simulink model "building_PHPP_carnot83"  (R2023b)
settings: Solver=ode23s  StartTime=-building.preruntime+8760*3600  StopTime=building.runtime+8760*3600  EnableMultiTasking=on
StartFcn:
  | tic
StopFcn:
  | toc
values from neighbouring files (symbols this model uses):
  building = obj    [BUILDING.m]    (also in create_building_automatic.m = building.save(); ini_building_automatic.m = building.add_variant_hvac(building.variant_hvac, hvac); load_building_automatic.m = building.save())
  cp = str2num(value)    [CONSTRUCTION.m]
  p = [timevec_weather weather(:,12)]    [BOUNDARY.m]    (also in WEATHER.m = 0; init_carnotUIBK.m = cell2mat(carnotUIBKpaths(i,2)))
  rho = str2num(value)    [CONSTRUCTION.m]    (also in theta_ground_v1.m = 2000)
undefined symbols (not defined in the file or in its folder): Dreifach, get_building, Qdot_C, Qdot_C_energy, Qdot_H, Qdot_H_energy, Qdot_I_electricity, Qdot_I_electricity_energy, Qdot_I_light, Qdot_I_light_energy, Qdot_I_person, Qdot_I_person_energy, Qdot_S, Qdot_S_energy, Qdot_T_ground, Qdot_T_ground_energy, Qdot_T_neighbour, Qdot_T_neighbour_energy, Qdot_T_opaque, Qdot_T_opaque_energy, Qdot_T_window, Qdot_T_window_energy, Qdot_V_infiltration, Qdot_V_infiltration_energy, Qdot_V_mech, Qdot_V_mech_energy, Qdot_V_window, Qdot_V_window_energy, Tc, Tr, Ts, Wärmeschutzglas, x_CO2, x_H2O, x_VOC
libraries: carnotUIBK x2418, carnot x1
(part 5 of 32)

== system building_PHPP_carnot83/BUILDING/INTERSECTION_7_9 ==
  AIB1 : Inport
  AIB2 : Inport  Port=2
  BDB1 : Inport  Port=3
  BDB2 : Inport  Port=4
  control : Inport  Port=5
  Bus Selector : BusSelector  OutputSignals=Qdot_S
  Bus Selector1 : BusSelector  OutputSignals=Qdot_S
  Subsystem : Subsystem
  Subsystem1 : Subsystem
  airexchange_1 : Subsystem  Variant=on  mask{zone=i.matrix_wd, window=1}
      mask prompts: window "wall"
      mask init: same as building_PHPP_carnot83/BUILDING/INTERSECTION_1_10/airexchange_1
      mask Display:
      | fprintf('AIR EXCHANGE\n')
      | %fprintf('\n%s', const.name)
  airexchange_2 : Subsystem  Variant=on  mask{zone=i.matrix_wd, window=2}
      mask prompts: window "wall"
      mask init: same as building_PHPP_carnot83/BUILDING/INTERSECTION_1_10/airexchange_1
      mask Display:
      | fprintf('AIR EXCHANGE\n')
      | %fprintf('\n%s', const.name)
  airexchange_3 : Subsystem  Variant=on  mask{zone=i.matrix_wd, window=3}
      mask prompts: window "wall"
      mask init: same as building_PHPP_carnot83/BUILDING/INTERSECTION_1_10/airexchange_1
      mask Display:
      | fprintf('AIR EXCHANGE\n')
      | %fprintf('\n%s', const.name)
  wall_1 : Subsystem  Variant=on  mask{zone=i.matrix_wd, construction=b.construction, wall=1}
      mask init: same as building_PHPP_carnot83/BUILDING/INTERSECTION_1_10/wall_1
      mask Display:
      | fprintf('CONSTRUCTION:\n')
      | fprintf('\n%s', const.name)
  wall_2 : Subsystem  Variant=on  mask{zone=i.matrix_wd, construction=b.construction, wall=2}
      mask init: same as building_PHPP_carnot83/BUILDING/INTERSECTION_1_10/wall_1
      mask Display:
      | fprintf('CONSTRUCTION:\n')
      | fprintf('\n%s', const.name)
  wall_3 : Subsystem  Variant=on  mask{zone=i.matrix_wd, construction=b.construction, wall=3}
      mask init: same as building_PHPP_carnot83/BUILDING/INTERSECTION_1_10/wall_1
      mask Display:
      | fprintf('CONSTRUCTION:\n')
      | fprintf('\n%s', const.name)
  S1 : Outport  VectorParamsAs1DForOutWhenUnconnected=off
  S2 : Outport  Port=2  VectorParamsAs1DForOutWhenUnconnected=off
  wires:
  BDB1/1 -> Bus Selector/1
  Bus Selector/1 -> wall_1/3(Qdot_sol1), wall_2/3(Qdot_sol1), wall_3/3(Qdot_sol1)  "<Qdot_S>"
  BDB2/1 -> Bus Selector1/1
  Bus Selector1/1 -> wall_1/4(Qdot_sol2), wall_2/4(Qdot_sol2), wall_3/4(Qdot_sol2)  "<Qdot_S>"
  control/1 -> airexchange_3/3(control), airexchange_2/3(control), airexchange_1/3(control)
  AIB2/1 -> wall_2/2(AIB2), wall_3/2(AIB2), airexchange_3/2(AIB2), airexchange_2/2(AIB2), airexchange_1/2(AIB2), wall_1/2(AIB2)
  AIB1/1 -> wall_2/1(AIB1), wall_3/1(AIB1), airexchange_3/1(AIB1), airexchange_2/1(AIB1), airexchange_1/1(AIB1), wall_1/1(AIB1)
  wall_1/1("[S1]") -> Subsystem/1(S1)
  wall_2/1("[S1]") -> Subsystem/2(S2)
  wall_3/1("[S1]") -> Subsystem/3(S3)
  airexchange_1/1("[S1]") -> Subsystem/4(S4)
  airexchange_2/1("[S1]") -> Subsystem/5(S5)
  airexchange_3/1("[S1]") -> Subsystem/6(S6)
  wall_1/2("[S2]") -> Subsystem1/1(S1)
  wall_2/2("[S2]") -> Subsystem1/2(S2)
  airexchange_3/2("[S2]") -> Subsystem1/6(S6)
  airexchange_2/2("[S2]") -> Subsystem1/5(S5)
  airexchange_1/2("[S2]") -> Subsystem1/4(S4)
  wall_3/2("[S2]") -> Subsystem1/3(S3)
  Subsystem/1(Sout) -> S1/1
  Subsystem1/1(Sout) -> S2/1

== system building_PHPP_carnot83/BUILDING/INTERSECTION_8_10 ==
  AIB1 : Inport
  AIB2 : Inport  Port=2
  BDB1 : Inport  Port=3
  BDB2 : Inport  Port=4
  control : Inport  Port=5
  Bus Selector : BusSelector  OutputSignals=Qdot_S
  Bus Selector1 : BusSelector  OutputSignals=Qdot_S
  Subsystem : Subsystem
  Subsystem1 : Subsystem
  airexchange_1 : Subsystem  Variant=on  mask{zone=i.matrix_wd, window=1}
      mask prompts: window "wall"
      mask init: same as building_PHPP_carnot83/BUILDING/INTERSECTION_1_10/airexchange_1
      mask Display:
      | fprintf('AIR EXCHANGE\n')
      | %fprintf('\n%s', const.name)
  airexchange_2 : Subsystem  Variant=on  mask{zone=i.matrix_wd, window=2}
      mask prompts: window "wall"
      mask init: same as building_PHPP_carnot83/BUILDING/INTERSECTION_1_10/airexchange_1
      mask Display:
      | fprintf('AIR EXCHANGE\n')
      | %fprintf('\n%s', const.name)
  airexchange_3 : Subsystem  Variant=on  mask{zone=i.matrix_wd, window=3}
      mask prompts: window "wall"
      mask init: same as building_PHPP_carnot83/BUILDING/INTERSECTION_1_10/airexchange_1
      mask Display:
      | fprintf('AIR EXCHANGE\n')
      | %fprintf('\n%s', const.name)
  wall_1 : Subsystem  Variant=on  mask{zone=i.matrix_wd, construction=b.construction, wall=1}
      mask init: same as building_PHPP_carnot83/BUILDING/INTERSECTION_1_10/wall_1
      mask Display:
      | fprintf('CONSTRUCTION:\n')
      | fprintf('\n%s', const.name)
  wall_2 : Subsystem  Variant=on  mask{zone=i.matrix_wd, construction=b.construction, wall=2}
      mask init: same as building_PHPP_carnot83/BUILDING/INTERSECTION_1_10/wall_1
      mask Display:
      | fprintf('CONSTRUCTION:\n')
      | fprintf('\n%s', const.name)
  wall_3 : Subsystem  Variant=on  mask{zone=i.matrix_wd, construction=b.construction, wall=3}
      mask init: same as building_PHPP_carnot83/BUILDING/INTERSECTION_1_10/wall_1
      mask Display:
      | fprintf('CONSTRUCTION:\n')
      | fprintf('\n%s', const.name)
  S1 : Outport  VectorParamsAs1DForOutWhenUnconnected=off
  S2 : Outport  Port=2  VectorParamsAs1DForOutWhenUnconnected=off
  wires:
  BDB1/1 -> Bus Selector/1
  Bus Selector/1 -> wall_1/3(Qdot_sol1), wall_2/3(Qdot_sol1), wall_3/3(Qdot_sol1)  "<Qdot_S>"
  BDB2/1 -> Bus Selector1/1
  Bus Selector1/1 -> wall_1/4(Qdot_sol2), wall_2/4(Qdot_sol2), wall_3/4(Qdot_sol2)  "<Qdot_S>"
  control/1 -> airexchange_3/3(control), airexchange_2/3(control), airexchange_1/3(control)
  AIB2/1 -> wall_2/2(AIB2), wall_3/2(AIB2), airexchange_3/2(AIB2), airexchange_2/2(AIB2), airexchange_1/2(AIB2), wall_1/2(AIB2)
  AIB1/1 -> wall_2/1(AIB1), wall_3/1(AIB1), airexchange_3/1(AIB1), airexchange_2/1(AIB1), airexchange_1/1(AIB1), wall_1/1(AIB1)
  wall_1/1("[S1]") -> Subsystem/1(S1)
  wall_2/1("[S1]") -> Subsystem/2(S2)
  wall_3/1("[S1]") -> Subsystem/3(S3)
  airexchange_1/1("[S1]") -> Subsystem/4(S4)
  airexchange_2/1("[S1]") -> Subsystem/5(S5)
  airexchange_3/1("[S1]") -> Subsystem/6(S6)
  wall_1/2("[S2]") -> Subsystem1/1(S1)
  wall_2/2("[S2]") -> Subsystem1/2(S2)
  airexchange_3/2("[S2]") -> Subsystem1/6(S6)
  airexchange_2/2("[S2]") -> Subsystem1/5(S5)
  airexchange_1/2("[S2]") -> Subsystem1/4(S4)
  wall_3/2("[S2]") -> Subsystem1/3(S3)
  Subsystem/1(Sout) -> S1/1
  Subsystem1/1(Sout) -> S2/1

== system building_PHPP_carnot83/BUILDING/INTERSECTION_8_9 ==
  AIB1 : Inport
  AIB2 : Inport  Port=2
  BDB1 : Inport  Port=3
  BDB2 : Inport  Port=4
  control : Inport  Port=5
  Bus Selector : BusSelector  OutputSignals=Qdot_S
  Bus Selector1 : BusSelector  OutputSignals=Qdot_S
  Subsystem : Subsystem
  Subsystem1 : Subsystem
  airexchange_1 : Subsystem  Variant=on  mask{zone=i.matrix_wd, window=1}
      mask prompts: window "wall"
      mask init: same as building_PHPP_carnot83/BUILDING/INTERSECTION_1_10/airexchange_1
      mask Display:
      | fprintf('AIR EXCHANGE\n')
      | %fprintf('\n%s', const.name)
  airexchange_2 : Subsystem  Variant=on  mask{zone=i.matrix_wd, window=2}
      mask prompts: window "wall"
      mask init: same as building_PHPP_carnot83/BUILDING/INTERSECTION_1_10/airexchange_1
      mask Display:
      | fprintf('AIR EXCHANGE\n')
      | %fprintf('\n%s', const.name)
  airexchange_3 : Subsystem  Variant=on  mask{zone=i.matrix_wd, window=3}
      mask prompts: window "wall"
      mask init: same as building_PHPP_carnot83/BUILDING/INTERSECTION_1_10/airexchange_1
      mask Display:
      | fprintf('AIR EXCHANGE\n')
      | %fprintf('\n%s', const.name)
  wall_1 : Subsystem  Variant=on  mask{zone=i.matrix_wd, construction=b.construction, wall=1}
      mask init: same as building_PHPP_carnot83/BUILDING/INTERSECTION_1_10/wall_1
      mask Display:
      | fprintf('CONSTRUCTION:\n')
      | fprintf('\n%s', const.name)
  wall_2 : Subsystem  Variant=on  mask{zone=i.matrix_wd, construction=b.construction, wall=2}
      mask init: same as building_PHPP_carnot83/BUILDING/INTERSECTION_1_10/wall_1
      mask Display:
      | fprintf('CONSTRUCTION:\n')
      | fprintf('\n%s', const.name)
  wall_3 : Subsystem  Variant=on  mask{zone=i.matrix_wd, construction=b.construction, wall=3}
      mask init: same as building_PHPP_carnot83/BUILDING/INTERSECTION_1_10/wall_1
      mask Display:
      | fprintf('CONSTRUCTION:\n')
      | fprintf('\n%s', const.name)
  S1 : Outport  VectorParamsAs1DForOutWhenUnconnected=off
  S2 : Outport  Port=2  VectorParamsAs1DForOutWhenUnconnected=off
  wires:
  BDB1/1 -> Bus Selector/1
  Bus Selector/1 -> wall_1/3(Qdot_sol1), wall_2/3(Qdot_sol1), wall_3/3(Qdot_sol1)  "<Qdot_S>"
  BDB2/1 -> Bus Selector1/1
  Bus Selector1/1 -> wall_1/4(Qdot_sol2), wall_2/4(Qdot_sol2), wall_3/4(Qdot_sol2)  "<Qdot_S>"
  control/1 -> airexchange_3/3(control), airexchange_2/3(control), airexchange_1/3(control)
  AIB2/1 -> wall_2/2(AIB2), wall_3/2(AIB2), airexchange_3/2(AIB2), airexchange_2/2(AIB2), airexchange_1/2(AIB2), wall_1/2(AIB2)
  AIB1/1 -> wall_2/1(AIB1), wall_3/1(AIB1), airexchange_3/1(AIB1), airexchange_2/1(AIB1), airexchange_1/1(AIB1), wall_1/1(AIB1)
  wall_1/1("[S1]") -> Subsystem/1(S1)
  wall_2/1("[S1]") -> Subsystem/2(S2)
  wall_3/1("[S1]") -> Subsystem/3(S3)
  airexchange_1/1("[S1]") -> Subsystem/4(S4)
  airexchange_2/1("[S1]") -> Subsystem/5(S5)
  airexchange_3/1("[S1]") -> Subsystem/6(S6)
  wall_1/2("[S2]") -> Subsystem1/1(S1)
  wall_2/2("[S2]") -> Subsystem1/2(S2)
  airexchange_3/2("[S2]") -> Subsystem1/6(S6)
  airexchange_2/2("[S2]") -> Subsystem1/5(S5)
  airexchange_1/2("[S2]") -> Subsystem1/4(S4)
  wall_3/2("[S2]") -> Subsystem1/3(S3)
  Subsystem/1(Sout) -> S1/1
  Subsystem1/1(Sout) -> S2/1

== system building_PHPP_carnot83/BUILDING/INTERSECTION_9_10 ==
  AIB1 : Inport
  AIB2 : Inport  Port=2
  BDB1 : Inport  Port=3
  BDB2 : Inport  Port=4
  control : Inport  Port=5
  Bus Selector : BusSelector  OutputSignals=Qdot_S
  Bus Selector1 : BusSelector  OutputSignals=Qdot_S
  Subsystem : Subsystem
  Subsystem1 : Subsystem
  airexchange_1 : Subsystem  Variant=on  mask{zone=i.matrix_wd, window=1}
      mask prompts: window "wall"
      mask init: same as building_PHPP_carnot83/BUILDING/INTERSECTION_1_10/airexchange_1
      mask Display:
      | fprintf('AIR EXCHANGE\n')
      | %fprintf('\n%s', const.name)
  airexchange_2 : Subsystem  Variant=on  mask{zone=i.matrix_wd, window=2}
      mask prompts: window "wall"
      mask init: same as building_PHPP_carnot83/BUILDING/INTERSECTION_1_10/airexchange_1
      mask Display:
      | fprintf('AIR EXCHANGE\n')
      | %fprintf('\n%s', const.name)
  airexchange_3 : Subsystem  Variant=on  mask{zone=i.matrix_wd, window=3}
      mask prompts: window "wall"
      mask init: same as building_PHPP_carnot83/BUILDING/INTERSECTION_1_10/airexchange_1
      mask Display:
      | fprintf('AIR EXCHANGE\n')
      | %fprintf('\n%s', const.name)
  wall_1 : Subsystem  Variant=on  mask{zone=i.matrix_wd, construction=b.construction, wall=1}
      mask init: same as building_PHPP_carnot83/BUILDING/INTERSECTION_1_10/wall_1
      mask Display:
      | fprintf('CONSTRUCTION:\n')
      | fprintf('\n%s', const.name)
  wall_2 : Subsystem  Variant=on  mask{zone=i.matrix_wd, construction=b.construction, wall=2}
      mask init: same as building_PHPP_carnot83/BUILDING/INTERSECTION_1_10/wall_1
      mask Display:
      | fprintf('CONSTRUCTION:\n')
      | fprintf('\n%s', const.name)
  wall_3 : Subsystem  Variant=on  mask{zone=i.matrix_wd, construction=b.construction, wall=3}
      mask init: same as building_PHPP_carnot83/BUILDING/INTERSECTION_1_10/wall_1
      mask Display:
      | fprintf('CONSTRUCTION:\n')
      | fprintf('\n%s', const.name)
  S1 : Outport  VectorParamsAs1DForOutWhenUnconnected=off
  S2 : Outport  Port=2  VectorParamsAs1DForOutWhenUnconnected=off
  wires:
  BDB1/1 -> Bus Selector/1
  Bus Selector/1 -> wall_1/3(Qdot_sol1), wall_2/3(Qdot_sol1), wall_3/3(Qdot_sol1)  "<Qdot_S>"
  BDB2/1 -> Bus Selector1/1
  Bus Selector1/1 -> wall_1/4(Qdot_sol2), wall_2/4(Qdot_sol2), wall_3/4(Qdot_sol2)  "<Qdot_S>"
  control/1 -> airexchange_3/3(control), airexchange_2/3(control), airexchange_1/3(control)
  AIB2/1 -> wall_2/2(AIB2), wall_3/2(AIB2), airexchange_3/2(AIB2), airexchange_2/2(AIB2), airexchange_1/2(AIB2), wall_1/2(AIB2)
  AIB1/1 -> wall_2/1(AIB1), wall_3/1(AIB1), airexchange_3/1(AIB1), airexchange_2/1(AIB1), airexchange_1/1(AIB1), wall_1/1(AIB1)
  wall_1/1("[S1]") -> Subsystem/1(S1)
  wall_2/1("[S1]") -> Subsystem/2(S2)
  wall_3/1("[S1]") -> Subsystem/3(S3)
  airexchange_1/1("[S1]") -> Subsystem/4(S4)
  airexchange_2/1("[S1]") -> Subsystem/5(S5)
  airexchange_3/1("[S1]") -> Subsystem/6(S6)
  wall_1/2("[S2]") -> Subsystem1/1(S1)
  wall_2/2("[S2]") -> Subsystem1/2(S2)
  airexchange_3/2("[S2]") -> Subsystem1/6(S6)
  airexchange_2/2("[S2]") -> Subsystem1/5(S5)
  airexchange_1/2("[S2]") -> Subsystem1/4(S4)
  wall_3/2("[S2]") -> Subsystem1/3(S3)
  Subsystem/1(Sout) -> S1/1
  Subsystem1/1(Sout) -> S2/1

== system building_PHPP_carnot83/BUILDING/Subsystem ==
  S1 : Inport
  S2 : Inport  Port=2
  S3 : Inport  Port=3
  S4 : Inport  Port=4
  S5 : Inport  Port=5
  S6 : Inport  Port=6
  S7 : Inport  Port=7
  S8 : Inport  Port=8
  S9 : Inport  Port=9
  S10 : Inport  Port=10
  S_initialize1 : carnotUIBK/general/S_initialize  SystemSampleTime=-1  VariantActivationTime=update diagram  AllowFlexibleInterface=on  Latency=0  AutoFrameSizeCalculation=off
  Ssum{,1..4} (5 alike) : carnotUIBK/general/Ssum  SystemSampleTime=-1  VariantActivationTime=update diagram  AllowFlexibleInterface=on  Latency=0  AutoFrameSizeCalculation=off
  Sout : Outport
  wires:
  S4/1 -> Ssum1/2
  S9/1 -> Ssum3/3
  Ssum1/1 -> Ssum2/1
  S10/1 -> Ssum4/2
  Ssum3/1 -> Ssum4/1
  Ssum2/1 -> Ssum3/1
  Ssum/1 -> Ssum1/1
  S5/1 -> Ssum1/3
  S1/1 -> Ssum/1
  Ssum4/1 -> Sout/1
  S8/1 -> Ssum3/2
  S2/1 -> Ssum/2
  S6/1 -> Ssum2/2
  S7/1 -> Ssum2/3
  S3/1 -> Ssum/3
  S_initialize1/1 -> Ssum4/3

== system building_PHPP_carnot83/BUILDING/Subsystem1 ==
  S1 : Inport
  S2 : Inport  Port=2
  S3 : Inport  Port=3
  S4 : Inport  Port=4
  S5 : Inport  Port=5
  S6 : Inport  Port=6
  S7 : Inport  Port=7
  S8 : Inport  Port=8
  S9 : Inport  Port=9
  S10 : Inport  Port=10
  S_initialize1 : carnotUIBK/general/S_initialize  SystemSampleTime=-1  VariantActivationTime=update diagram  AllowFlexibleInterface=on  Latency=0  AutoFrameSizeCalculation=off
  Ssum{,1..4} (5 alike) : carnotUIBK/general/Ssum  SystemSampleTime=-1  VariantActivationTime=update diagram  AllowFlexibleInterface=on  Latency=0  AutoFrameSizeCalculation=off
  Sout : Outport
  wires:
  S_initialize1/1 -> Ssum4/3
  S3/1 -> Ssum/3
  S7/1 -> Ssum2/3
  S6/1 -> Ssum2/2
  S2/1 -> Ssum/2
  S8/1 -> Ssum3/2
  Ssum4/1 -> Sout/1
  S1/1 -> Ssum/1
  S5/1 -> Ssum1/3
  Ssum/1 -> Ssum1/1
  Ssum2/1 -> Ssum3/1
  Ssum3/1 -> Ssum4/1
  S10/1 -> Ssum4/2
  Ssum1/1 -> Ssum2/1
  S9/1 -> Ssum3/3
  S4/1 -> Ssum1/2

== system building_PHPP_carnot83/BUILDING/Subsystem2 ==
  S1 : Inport
  S2 : Inport  Port=2
  S3 : Inport  Port=3
  S4 : Inport  Port=4
  S5 : Inport  Port=5
  S6 : Inport  Port=6
  S7 : Inport  Port=7
  S8 : Inport  Port=8
  S9 : Inport  Port=9
  S10 : Inport  Port=10
  S_initialize1 : carnotUIBK/general/S_initialize  SystemSampleTime=-1  VariantActivationTime=update diagram  AllowFlexibleInterface=on  Latency=0  AutoFrameSizeCalculation=off
  Ssum{,1..4} (5 alike) : carnotUIBK/general/Ssum  SystemSampleTime=-1  VariantActivationTime=update diagram  AllowFlexibleInterface=on  Latency=0  AutoFrameSizeCalculation=off
  Sout : Outport
  wires:
  S4/1 -> Ssum1/2
  S9/1 -> Ssum3/3
  Ssum1/1 -> Ssum2/1
  S10/1 -> Ssum4/2
  Ssum3/1 -> Ssum4/1
  Ssum2/1 -> Ssum3/1
  Ssum/1 -> Ssum1/1
  S5/1 -> Ssum1/3
  S1/1 -> Ssum/1
  Ssum4/1 -> Sout/1
  S8/1 -> Ssum3/2
  S2/1 -> Ssum/2
  S6/1 -> Ssum2/2
  S7/1 -> Ssum2/3
  S3/1 -> Ssum/3
  S_initialize1/1 -> Ssum4/3

== system building_PHPP_carnot83/BUILDING/Subsystem3 ==
  S1 : Inport
  S2 : Inport  Port=2
  S3 : Inport  Port=3
  S4 : Inport  Port=4
  S5 : Inport  Port=5
  S6 : Inport  Port=6
  S7 : Inport  Port=7
  S8 : Inport  Port=8
  S9 : Inport  Port=9
  S10 : Inport  Port=10
  S_initialize1 : carnotUIBK/general/S_initialize  SystemSampleTime=-1  VariantActivationTime=update diagram  AllowFlexibleInterface=on  Latency=0  AutoFrameSizeCalculation=off
  Ssum{,1..4} (5 alike) : carnotUIBK/general/Ssum  SystemSampleTime=-1  VariantActivationTime=update diagram  AllowFlexibleInterface=on  Latency=0  AutoFrameSizeCalculation=off
  Sout : Outport
  wires:
  S_initialize1/1 -> Ssum4/3
  S3/1 -> Ssum/3
  S7/1 -> Ssum2/3
  S6/1 -> Ssum2/2
  S2/1 -> Ssum/2
  S8/1 -> Ssum3/2
  Ssum4/1 -> Sout/1
  S1/1 -> Ssum/1
  S5/1 -> Ssum1/3
  Ssum/1 -> Ssum1/1
  Ssum2/1 -> Ssum3/1
  Ssum3/1 -> Ssum4/1
  S10/1 -> Ssum4/2
  Ssum1/1 -> Ssum2/1
  S9/1 -> Ssum3/3
  S4/1 -> Ssum1/2

== system building_PHPP_carnot83/BUILDING/Subsystem4 ==
  S1 : Inport
  S2 : Inport  Port=2
  S3 : Inport  Port=3
  S4 : Inport  Port=4
  S5 : Inport  Port=5
  S6 : Inport  Port=6
  S7 : Inport  Port=7
  S8 : Inport  Port=8
  S9 : Inport  Port=9
  S10 : Inport  Port=10
  S_initialize1 : carnotUIBK/general/S_initialize  SystemSampleTime=-1  VariantActivationTime=update diagram  AllowFlexibleInterface=on  Latency=0  AutoFrameSizeCalculation=off
  Ssum{,1..4} (5 alike) : carnotUIBK/general/Ssum  SystemSampleTime=-1  VariantActivationTime=update diagram  AllowFlexibleInterface=on  Latency=0  AutoFrameSizeCalculation=off
  Sout : Outport
  wires:
  S4/1 -> Ssum1/2
  S9/1 -> Ssum3/3
  Ssum1/1 -> Ssum2/1
  S10/1 -> Ssum4/2
  Ssum3/1 -> Ssum4/1
  Ssum2/1 -> Ssum3/1
  Ssum/1 -> Ssum1/1
  S5/1 -> Ssum1/3
  S1/1 -> Ssum/1
  Ssum4/1 -> Sout/1
  S8/1 -> Ssum3/2
  S2/1 -> Ssum/2
  S6/1 -> Ssum2/2
  S7/1 -> Ssum2/3
  S3/1 -> Ssum/3
  S_initialize1/1 -> Ssum4/3

== system building_PHPP_carnot83/BUILDING/Subsystem5 ==
  S1 : Inport
  S2 : Inport  Port=2
  S3 : Inport  Port=3
  S4 : Inport  Port=4
  S5 : Inport  Port=5
  S6 : Inport  Port=6
  S7 : Inport  Port=7
  S8 : Inport  Port=8
  S9 : Inport  Port=9
  S10 : Inport  Port=10
  S_initialize1 : carnotUIBK/general/S_initialize  SystemSampleTime=-1  VariantActivationTime=update diagram  AllowFlexibleInterface=on  Latency=0  AutoFrameSizeCalculation=off
  Ssum{,1..4} (5 alike) : carnotUIBK/general/Ssum  SystemSampleTime=-1  VariantActivationTime=update diagram  AllowFlexibleInterface=on  Latency=0  AutoFrameSizeCalculation=off
  Sout : Outport
  wires:
  S_initialize1/1 -> Ssum4/3
  S3/1 -> Ssum/3
  S7/1 -> Ssum2/3
  S6/1 -> Ssum2/2
  S2/1 -> Ssum/2
  S8/1 -> Ssum3/2
  Ssum4/1 -> Sout/1
  S1/1 -> Ssum/1
  S5/1 -> Ssum1/3
  Ssum/1 -> Ssum1/1
  Ssum2/1 -> Ssum3/1
  Ssum3/1 -> Ssum4/1
  S10/1 -> Ssum4/2
  Ssum1/1 -> Ssum2/1
  S9/1 -> Ssum3/3
  S4/1 -> Ssum1/2

== system building_PHPP_carnot83/BUILDING/Subsystem6 ==
  S1 : Inport
  S2 : Inport  Port=2
  S3 : Inport  Port=3
  S4 : Inport  Port=4
  S5 : Inport  Port=5
  S6 : Inport  Port=6
  S7 : Inport  Port=7
  S8 : Inport  Port=8
  S9 : Inport  Port=9
  S10 : Inport  Port=10
  S_initialize1 : carnotUIBK/general/S_initialize  SystemSampleTime=-1  VariantActivationTime=update diagram  AllowFlexibleInterface=on  Latency=0  AutoFrameSizeCalculation=off
  Ssum{,1..4} (5 alike) : carnotUIBK/general/Ssum  SystemSampleTime=-1  VariantActivationTime=update diagram  AllowFlexibleInterface=on  Latency=0  AutoFrameSizeCalculation=off
  Sout : Outport
  wires:
  S4/1 -> Ssum1/2
  S9/1 -> Ssum3/3
  Ssum1/1 -> Ssum2/1
  S10/1 -> Ssum4/2
  Ssum3/1 -> Ssum4/1
  Ssum2/1 -> Ssum3/1
  Ssum/1 -> Ssum1/1
  S5/1 -> Ssum1/3
  S1/1 -> Ssum/1
  Ssum4/1 -> Sout/1
  S8/1 -> Ssum3/2
  S2/1 -> Ssum/2
  S6/1 -> Ssum2/2
  S7/1 -> Ssum2/3
  S3/1 -> Ssum/3
  S_initialize1/1 -> Ssum4/3

== system building_PHPP_carnot83/BUILDING/Subsystem7 ==
  S1 : Inport
  S2 : Inport  Port=2
  S3 : Inport  Port=3
  S4 : Inport  Port=4
  S5 : Inport  Port=5
  S6 : Inport  Port=6
  S7 : Inport  Port=7
  S8 : Inport  Port=8
  S9 : Inport  Port=9
  S10 : Inport  Port=10
  S_initialize1 : carnotUIBK/general/S_initialize  SystemSampleTime=-1  VariantActivationTime=update diagram  AllowFlexibleInterface=on  Latency=0  AutoFrameSizeCalculation=off
  Ssum{,1..4} (5 alike) : carnotUIBK/general/Ssum  SystemSampleTime=-1  VariantActivationTime=update diagram  AllowFlexibleInterface=on  Latency=0  AutoFrameSizeCalculation=off
  Sout : Outport
  wires:
  S_initialize1/1 -> Ssum4/3
  S3/1 -> Ssum/3
  S7/1 -> Ssum2/3
  S6/1 -> Ssum2/2
  S2/1 -> Ssum/2
  S8/1 -> Ssum3/2
  Ssum4/1 -> Sout/1
  S1/1 -> Ssum/1
  S5/1 -> Ssum1/3
  Ssum/1 -> Ssum1/1
  Ssum2/1 -> Ssum3/1
  Ssum3/1 -> Ssum4/1
  S10/1 -> Ssum4/2
  Ssum1/1 -> Ssum2/1
  S9/1 -> Ssum3/3
  S4/1 -> Ssum1/2

== system building_PHPP_carnot83/BUILDING/Subsystem8 ==
  S1 : Inport
  S2 : Inport  Port=2
  S3 : Inport  Port=3
  S4 : Inport  Port=4
  S5 : Inport  Port=5
  S6 : Inport  Port=6
  S7 : Inport  Port=7
  S8 : Inport  Port=8
  S9 : Inport  Port=9
  S10 : Inport  Port=10
  S_initialize1 : carnotUIBK/general/S_initialize  SystemSampleTime=-1  VariantActivationTime=update diagram  AllowFlexibleInterface=on  Latency=0  AutoFrameSizeCalculation=off
  Ssum{,1..4} (5 alike) : carnotUIBK/general/Ssum  SystemSampleTime=-1  VariantActivationTime=update diagram  AllowFlexibleInterface=on  Latency=0  AutoFrameSizeCalculation=off
  Sout : Outport
  wires:
  S4/1 -> Ssum1/2
  S9/1 -> Ssum3/3
  Ssum1/1 -> Ssum2/1
  S10/1 -> Ssum4/2
  Ssum3/1 -> Ssum4/1
  Ssum2/1 -> Ssum3/1
  Ssum/1 -> Ssum1/1
  S5/1 -> Ssum1/3
  S1/1 -> Ssum/1
  Ssum4/1 -> Sout/1
  S8/1 -> Ssum3/2
  S2/1 -> Ssum/2
  S6/1 -> Ssum2/2
  S7/1 -> Ssum2/3
  S3/1 -> Ssum/3
  S_initialize1/1 -> Ssum4/3

== system building_PHPP_carnot83/BUILDING/Subsystem9 ==
  S1 : Inport
  S2 : Inport  Port=2
  S3 : Inport  Port=3
  S4 : Inport  Port=4
  S5 : Inport  Port=5
  S6 : Inport  Port=6
  S7 : Inport  Port=7
  S8 : Inport  Port=8
  S9 : Inport  Port=9
  S10 : Inport  Port=10
  S_initialize1 : carnotUIBK/general/S_initialize  SystemSampleTime=-1  VariantActivationTime=update diagram  AllowFlexibleInterface=on  Latency=0  AutoFrameSizeCalculation=off
  Ssum{,1..4} (5 alike) : carnotUIBK/general/Ssum  SystemSampleTime=-1  VariantActivationTime=update diagram  AllowFlexibleInterface=on  Latency=0  AutoFrameSizeCalculation=off
  Sout : Outport
  wires:
  S_initialize1/1 -> Ssum4/3
  S3/1 -> Ssum/3
  S7/1 -> Ssum2/3
  S6/1 -> Ssum2/2
  S2/1 -> Ssum/2
  S8/1 -> Ssum3/2
  Ssum4/1 -> Sout/1
  S1/1 -> Ssum/1
  S5/1 -> Ssum1/3
  Ssum/1 -> Ssum1/1
  Ssum2/1 -> Ssum3/1
  Ssum3/1 -> Ssum4/1
  S10/1 -> Ssum4/2
  Ssum1/1 -> Ssum2/1
  S9/1 -> Ssum3/3
  S4/1 -> Ssum1/2

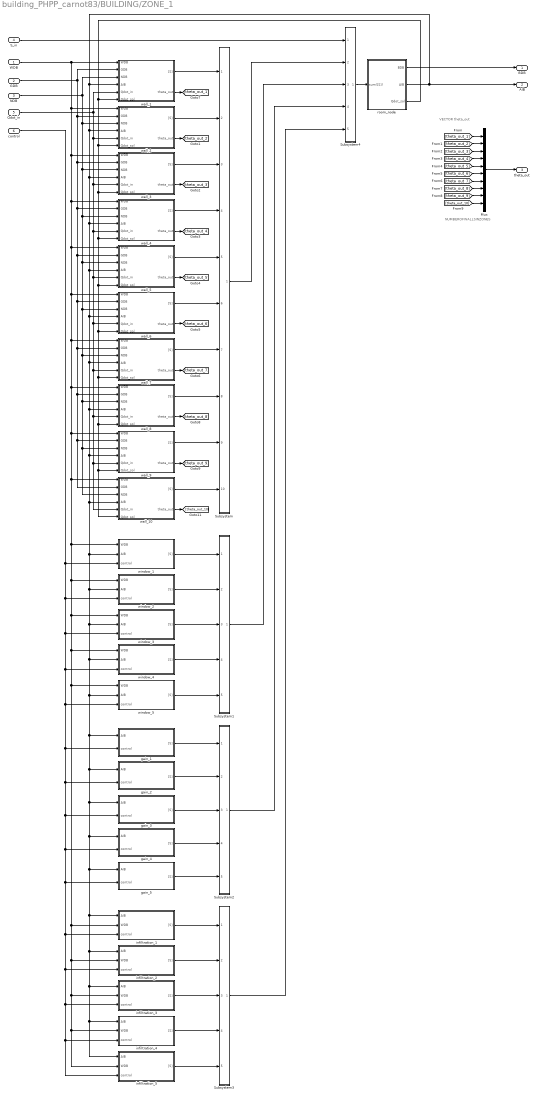
== system building_PHPP_carnot83/BUILDING/ZONE_1 ==
  note: VECTOR theta_out
  note: NUMBEROFWALLSINZONES
  WDB : Inport
  GDB : Inport  Port=2
  NDB : Inport  Port=3
  S_in : Inport  Port=4
  Qdot_in : Inport  Port=5
  control : Inport  Port=6
  Mux : Mux  Inputs=10
  Subsystem : Subsystem
  Subsystem1 : Subsystem
  Subsystem2 : Subsystem
  Subsystem3 : Subsystem
  Subsystem4 : Subsystem
  gain_1 : Subsystem  Variant=on  mask{zone=z.matrix_gains, gains=b.gains, subgain=1}
      mask init:
      | if (subgain <= size(zone,1))
      |     ga = gains.get_gain(zone{subgain,1});
      |     
      |     type = zone{subgain,3};
      |     timevalues = zone{subgain,4};
      |     timeduration = zone{subgain,5};
      |     values1 = zone{subgain,6};
      |     values2 = zone{subgain,7};
      |     values3 = zone{subgain,8};
      |     control = zone{subgain,9};
      | else
      |     ga.name = 'no gains';
      |     
      |     type = 0;
      |     timevalues = [0 1 24]*3600;
      |     timeduration = [1 23]*3600;
      |     values1 = [0 0];
      |     values2 = [0 0];
      |     values3 = [0 0];
      |     control = 1;
      | end
      mask Display:
      | fprintf('GAINS:\n')
      | fprintf('\n%s', ga.name)
  gain_2 : Subsystem  Variant=on  mask{zone=z.matrix_gains, gains=b.gains, subgain=2}
      mask init: same as building_PHPP_carnot83/BUILDING/ZONE_1/gain_1
      mask Display:
      | fprintf('GAINS:\n')
      | fprintf('\n%s', ga.name)
  gain_3 : Subsystem  Variant=on  mask{zone=z.matrix_gains, gains=b.gains, subgain=3}
      mask init: same as building_PHPP_carnot83/BUILDING/ZONE_1/gain_1
      mask Display:
      | fprintf('GAINS:\n')
      | fprintf('\n%s', ga.name)
  gain_4 : Subsystem  Variant=on  mask{zone=z.matrix_gains, gains=b.gains, subgain=4}
      mask init: same as building_PHPP_carnot83/BUILDING/ZONE_1/gain_1
      mask Display:
      | fprintf('GAINS:\n')
      | fprintf('\n%s', ga.name)
  gain_5 : Subsystem  Variant=on  mask{zone=z.matrix_gains, gains=b.gains, subgain=4}
      mask init: same as building_PHPP_carnot83/BUILDING/ZONE_1/gain_1
      mask Display:
      | fprintf('GAINS:\n')
      | fprintf('\n%s', ga.name)
  infiltration_1 : Subsystem  Variant=on  mask{zone=z.matrix_wi, window=1}
      mask init:
      | if (window <= size(zone,1))
      |     window_width = zone{window,2};
      |     window_height = zone{window,3};
      |     window_z = zone{window,20};
      |     inf_C = zone{window,21};
      |     inf_n = zone{window,22};
      |     inf_V = zone{window,23};
      |     control = zone{window,24};
      | else
      |     window_width = 0;
      |     window_height = 0;
      |     window_z = 0;
      |     inf_C = [0 0 0];
      |     inf_n = [0 0 0];
      |     inf_V = [0 0 0];
      |     control = 1;
      | end
      mask Display:
      | fprintf('INFILTRATION:\n')
      | %fprintf('\n%s', const.name)
  infiltration_2 : Subsystem  Variant=on  mask{zone=z.matrix_wi, window=2}
      mask init: same as building_PHPP_carnot83/BUILDING/ZONE_1/infiltration_1
      mask Display:
      | fprintf('INFILTRATION:\n')
      | %fprintf('\n%s', const.name)
  infiltration_3 : Subsystem  Variant=on  mask{zone=z.matrix_wi, window=3}
      mask init: same as building_PHPP_carnot83/BUILDING/ZONE_1/infiltration_1
      mask Display:
      | fprintf('INFILTRATION:\n')
      | %fprintf('\n%s', const.name)
  infiltration_4 : Subsystem  Variant=on  mask{zone=z.matrix_wi, window=4}
      mask init: same as building_PHPP_carnot83/BUILDING/ZONE_1/infiltration_1
      mask Display:
      | fprintf('INFILTRATION:\n')
      | %fprintf('\n%s', const.name)
  infiltration_5 : Subsystem  Variant=on  mask{zone=z.matrix_wi, window=5}
      mask init: same as building_PHPP_carnot83/BUILDING/ZONE_1/infiltration_1
      mask Display:
      | fprintf('INFILTRATION:\n')
      | %fprintf('\n%s', const.name)
  room_node : Subsystem  Variant=on
  wall_1 : Subsystem  Variant=on  mask{zone=z.matrix_wd, construction=b.construction, wall=1}
      mask init:
      | if (wall <= size(zone,1))
      |     const = construction.get_structure(zone(wall,1));
      |     wallsurface = zone{wall,2};
      |     pos = [zone{wall,4} zone{wall,5} zone{wall,6}];
      |     view_factor = zone{wall,9};
      |     amb_factor = zone{wall,10};
      |     solar_ratio = zone{wall,11};
      |     boundary = zone{wall,12};
      |     % still to be implemented with ENABLE, not a VARIANT!
      |     model_ht = zone{wall,8};
      | else
      |     const.name = 'no construction';
      |     wallsurface = 0;
      |     pos = [0 0 0];
      |     view_factor = 0;
      |     amb_factor = 0;
      |     solar_ratio = 0;
      |     boundary = 0;
      |     model_ht = 0;
      | end
      mask Display:
      | fprintf('CONSTRUCTION:\n')
      | fprintf('\n%s', const.name)
  wall_10 : Subsystem  Variant=on  mask{zone=z.matrix_wd, construction=b.construction, wall=10}
      mask init: same as building_PHPP_carnot83/BUILDING/ZONE_1/wall_1
      mask Display:
      | fprintf('CONSTRUCTION:\n')
      | fprintf('\n%s', const.name)
  wall_2 : Subsystem  Variant=on  mask{zone=z.matrix_wd, construction=b.construction, wall=2}
      mask init: same as building_PHPP_carnot83/BUILDING/ZONE_1/wall_1
      mask Display:
      | fprintf('CONSTRUCTION:\n')
      | fprintf('\n%s', const.name)
  wall_3 : Subsystem  Variant=on  mask{zone=z.matrix_wd, construction=b.construction, wall=3}
      mask init: same as building_PHPP_carnot83/BUILDING/ZONE_1/wall_1
      mask Display:
      | fprintf('CONSTRUCTION:\n')
      | fprintf('\n%s', const.name)
  wall_4 : Subsystem  Variant=on  mask{zone=z.matrix_wd, construction=b.construction, wall=4}
      mask init: same as building_PHPP_carnot83/BUILDING/ZONE_1/wall_1
      mask Display:
      | fprintf('CONSTRUCTION:\n')
      | fprintf('\n%s', const.name)
  wall_5 : Subsystem  Variant=on  mask{zone=z.matrix_wd, construction=b.construction, wall=5}
      mask init: same as building_PHPP_carnot83/BUILDING/ZONE_1/wall_1
      mask Display:
      | fprintf('CONSTRUCTION:\n')
      | fprintf('\n%s', const.name)
  wall_6 : Subsystem  Variant=on  mask{zone=z.matrix_wd, construction=b.construction, wall=6}
      mask init: same as building_PHPP_carnot83/BUILDING/ZONE_1/wall_1
      mask Display:
      | fprintf('CONSTRUCTION:\n')
      | fprintf('\n%s', const.name)
  wall_7 : Subsystem  Variant=on  mask{zone=z.matrix_wd, construction=b.construction, wall=7}
      mask init: same as building_PHPP_carnot83/BUILDING/ZONE_1/wall_1
      mask Display:
      | fprintf('CONSTRUCTION:\n')
      | fprintf('\n%s', const.name)
  wall_8 : Subsystem  Variant=on  mask{zone=z.matrix_wd, construction=b.construction, wall=8}
      mask init: same as building_PHPP_carnot83/BUILDING/ZONE_1/wall_1
      mask Display:
      | fprintf('CONSTRUCTION:\n')
      | fprintf('\n%s', const.name)
  wall_9 : Subsystem  Variant=on  mask{zone=z.matrix_wd, construction=b.construction, wall=9}
      mask init: same as building_PHPP_carnot83/BUILDING/ZONE_1/wall_1
      mask Display:
      | fprintf('CONSTRUCTION:\n')
      | fprintf('\n%s', const.name)
  window_1 : Subsystem  Variant=on  mask{zone=z.matrix_wi, construction=b.construction, window=1}
      mask init:
      | if (window <= size(zone,1))
      |     const = construction.get_structure(zone(window,1));
      |     
      |     window_width = zone{window,2};
      |     window_heigth = zone{window,3};
      |     windowsurface = window_heigth*window_width;
      |     glassurface = zone{window,10};
      |     Psi_installation = zone{window,16};
      |     l_glas = zone{window,17};
      |     pos = [zone{window,5} zone{window,6} zone{window,7}];
      |     view_factor = zone{window,11};
      |     amb_factor = zone{window,12};
      |     r_frame = zone{window,9};
      |     control = zone{window,18};
      |     
      |     % calculation u-value
      | %     const.parameter.U_g*glassurface
      | %     const.parameter.U_f*(windowsurface-glassurface)
      | %     const.parameter.psi_ge*l_glas
      | %     Psi_installation
      |     UA = const.parameter.U_g*glassurface + const.parameter.U_f*(windowsurface-glassurface)+const.parameter.psi_ge*l_glas+Psi_installation;
      |     Uvalue = UA / windowsurface;
      |     
      | else
      |     const.name = 'no construction';
      |     
      |     window_width = 0;
      |     window_heigth = 0;
      |     windowsurface = window_heigth*window_width;
      |     glassurface = 0;
      |     Psi_installation = 0;
      |     l_glas = 0;
      |     pos = [0 0 0];
      |     view_factor = 0;
      |     amb_factor = 0;
      |     r_frame = 0;
      |     control = 1;
      |     
      |     UA = 0;
      |     Uvalue = 0;
      | end
      mask Display:
      | fprintf('CONSTRUCTION:\n')
      | fprintf('\n%s', const.name)
  window_2 : Subsystem  Variant=on  mask{zone=z.matrix_wi, construction=b.construction, window=2}
      mask init: same as building_PHPP_carnot83/BUILDING/ZONE_1/window_1
      mask Display:
      | fprintf('CONSTRUCTION:\n')
      | fprintf('\n%s', const.name)
  window_3 : Subsystem  Variant=on  mask{zone=z.matrix_wi, construction=b.construction, window=3}
      mask init: same as building_PHPP_carnot83/BUILDING/ZONE_1/window_1
      mask Display:
      | fprintf('CONSTRUCTION:\n')
      | fprintf('\n%s', const.name)
  window_4 : Subsystem  Variant=on  mask{zone=z.matrix_wi, construction=b.construction, window=4}
      mask init: same as building_PHPP_carnot83/BUILDING/ZONE_1/window_1
      mask Display:
      | fprintf('CONSTRUCTION:\n')
      | fprintf('\n%s', const.name)
  window_5 : Subsystem  Variant=on  mask{zone=z.matrix_wi, construction=b.construction, window=5}
      mask init: same as building_PHPP_carnot83/BUILDING/ZONE_1/window_1
      mask Display:
      | fprintf('CONSTRUCTION:\n')
      | fprintf('\n%s', const.name)
  BDB : Outport  VectorParamsAs1DForOutWhenUnconnected=off
  AIB : Outport  Port=2  VectorParamsAs1DForOutWhenUnconnected=off
  theta_out : Outport  Port=3  VectorParamsAs1DForOutWhenUnconnected=off
  wires:
  room_node/1(BDB) -> BDB/1
  S_in/1 -> Subsystem4/1(S1)
  Qdot_in/1 -> wall_1/5(Qdot_in), wall_3/5(Qdot_in), wall_4/5(Qdot_in), wall_10/5(Qdot_in), wall_9/5(Qdot_in), wall_8/5(Qdot_in), wall_7/5(Qdot_in), wall_6/5(Qdot_in), wall_5/5(Qdot_in), wall_2/5(Qdot_in)
  Subsystem4/1(Sout) -> room_node/1(sum([S]))
  room_node/3(Qdot_sol) -> wall_3/6(Qdot_sol), wall_4/6(Qdot_sol), wall_6/6(Qdot_sol), wall_8/6(Qdot_sol), wall_10/6(Qdot_sol), wall_9/6(Qdot_sol), wall_7/6(Qdot_sol), wall_5/6(Qdot_sol), wall_2/6(Qdot_sol), wall_1/6(Qdot_sol)
  wall_1/2(theta_out) -> [theta_out_1]
  control/1 -> gain_2/2(control), gain_3/2(control), infiltration_1/3(control), infiltration_2/3(control), infiltration_3/3(control), infiltration_4/3(control), infiltration_5/3(control), gain_5/2(control), gain_4/2(control), gain_1/2(control), window_5/3(control), window_4/3(control), window_3/3(control), window_2/3(control), window_1/3(control)
  Mux/1 -> theta_out/1
  [theta_out_1] -> Mux/1
  [theta_out_2] -> Mux/2
  [theta_out_10] -> Mux/10
  [theta_out_9] -> Mux/9
  [theta_out_8] -> Mux/8
  [theta_out_7] -> Mux/7
  [theta_out_6] -> Mux/6
  [theta_out_5] -> Mux/5
  [theta_out_4] -> Mux/4
  [theta_out_3] -> Mux/3
  wall_2/2(theta_out) -> [theta_out_2]
  GDB/1 -> wall_1/2(GDB), wall_3/2(GDB), wall_4/2(GDB), wall_6/2(GDB), wall_8/2(GDB), wall_10/2(GDB), wall_9/2(GDB), wall_7/2(GDB), wall_5/2(GDB), wall_2/2(GDB)
  wall_3/2(theta_out) -> [theta_out_3]
  wall_4/2(theta_out) -> [theta_out_4]
  wall_5/2(theta_out) -> [theta_out_5]
  wall_6/2(theta_out) -> [theta_out_6]
  NDB/1 -> wall_1/3(NDB), wall_3/3(NDB), wall_4/3(NDB), wall_6/3(NDB), wall_10/3(NDB), wall_9/3(NDB), wall_8/3(NDB), wall_7/3(NDB), wall_5/3(NDB), wall_2/3(NDB)
  Subsystem/1(Sout) -> Subsystem4/2(S2)
  window_1/1("[S]") -> Subsystem1/1(S1)
  window_5/1("[S]") -> Subsystem1/5(S5)
  window_2/1("[S]") -> Subsystem1/2(S2)
  window_3/1("[S]") -> Subsystem1/3(S3)
  window_4/1("[S]") -> Subsystem1/4(S4)
  Subsystem1/1(Sout) -> Subsystem4/3(S3)
  gain_1/1("[S]") -> Subsystem2/1(S1)
  gain_5/1("[S]") -> Subsystem2/5(S5)
  gain_2/1("[S]") -> Subsystem2/2(S2)
  gain_3/1("[S]") -> Subsystem2/3(S3)
  gain_4/1("[S]") -> Subsystem2/4(S4)
  Subsystem2/1(Sout) -> Subsystem4/4(S4)
  infiltration_1/1("[S]") -> Subsystem3/1(S1)
  infiltration_5/1("[S]") -> Subsystem3/5(S5)
  infiltration_4/1("[S]") -> Subsystem3/4(S4)
  infiltration_3/1("[S]") -> Subsystem3/3(S3)
  infiltration_2/1("[S]") -> Subsystem3/2(S2)
  Subsystem3/1(Sout) -> Subsystem4/5(S5)
  WDB/1 -> wall_3/1(WDB), wall_4/1(WDB), wall_5/1(WDB), wall_6/1(WDB), wall_7/1(WDB), wall_8/1(WDB), wall_10/1(WDB), window_1/1(WDB), window_4/1(WDB), infiltration_2/2(WDB), infiltration_3/2(WDB), infiltration_4/2(WDB), infiltration_5/2(WDB), infiltration_1/2(WDB), window_5/1(WDB), window_3/1(WDB), window_2/1(WDB), wall_9/1(WDB), wall_2/1(WDB), wall_1/1(WDB)
  room_node/2(AIB) -> AIB/1, wall_3/4(AIB), wall_4/4(AIB), wall_5/4(AIB), wall_6/4(AIB), wall_7/4(AIB), wall_8/4(AIB), wall_9/4(AIB), wall_10/4(AIB), gain_2/1(AIB), gain_3/1(AIB), infiltration_2/1(AIB), infiltration_3/1(AIB), infiltration_4/1(AIB), infiltration_5/1(AIB), infiltration_1/1(AIB), gain_5/1(AIB), gain_4/1(AIB), gain_1/1(AIB), window_5/2(AIB), window_4/2(AIB), window_3/2(AIB), window_2/2(AIB), window_1/2(AIB), wall_2/4(AIB), wall_1/4(AIB)
  wall_7/2(theta_out) -> [theta_out_7]
  wall_8/2(theta_out) -> [theta_out_8]
  wall_9/2(theta_out) -> [theta_out_9]
  wall_10/2(theta_out) -> [theta_out_10]
  wall_1/1("[S]") -> Subsystem/1(S1)
  wall_2/1("[S]") -> Subsystem/2(S2)
  wall_3/1("[S]") -> Subsystem/3(S3)
  wall_4/1("[S]") -> Subsystem/4(S4)
  wall_5/1("[S]") -> Subsystem/5(S5)
  wall_6/1("[S]") -> Subsystem/6(S6)
  wall_7/1("[S]") -> Subsystem/7(S7)
  wall_8/1("[S]") -> Subsystem/8(S8)
  wall_9/1("[S]") -> Subsystem/9(S9)
  wall_10/1("[S]") -> Subsystem/10(S10)

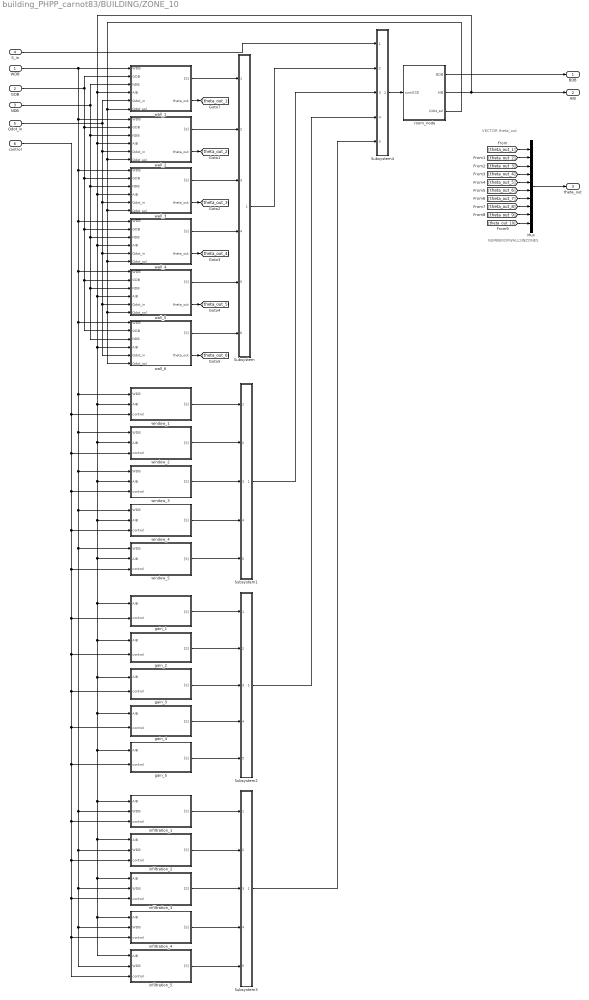
== system building_PHPP_carnot83/BUILDING/ZONE_10 ==
  note: VECTOR theta_out
  note: NUMBEROFWALLSINZONES
  WDB : Inport
  GDB : Inport  Port=2
  NDB : Inport  Port=3
  S_in : Inport  Port=4
  Qdot_in : Inport  Port=5
  control : Inport  Port=6
  Mux : Mux  Inputs=10
  Subsystem : Subsystem
  Subsystem1 : Subsystem
  Subsystem2 : Subsystem
  Subsystem3 : Subsystem
  Subsystem4 : Subsystem
  gain_1 : Subsystem  Variant=on  mask{zone=z.matrix_gains, gains=b.gains, subgain=1}
      mask init: same as building_PHPP_carnot83/BUILDING/ZONE_1/gain_1
      mask Display:
      | fprintf('GAINS:\n')
      | fprintf('\n%s', ga.name)
  gain_2 : Subsystem  Variant=on  mask{zone=z.matrix_gains, gains=b.gains, subgain=2}
      mask init: same as building_PHPP_carnot83/BUILDING/ZONE_1/gain_1
      mask Display:
      | fprintf('GAINS:\n')
      | fprintf('\n%s', ga.name)
  gain_3 : Subsystem  Variant=on  mask{zone=z.matrix_gains, gains=b.gains, subgain=3}
      mask init: same as building_PHPP_carnot83/BUILDING/ZONE_1/gain_1
      mask Display:
      | fprintf('GAINS:\n')
      | fprintf('\n%s', ga.name)
  gain_4 : Subsystem  Variant=on  mask{zone=z.matrix_gains, gains=b.gains, subgain=4}
      mask init: same as building_PHPP_carnot83/BUILDING/ZONE_1/gain_1
      mask Display:
      | fprintf('GAINS:\n')
      | fprintf('\n%s', ga.name)
  gain_5 : Subsystem  Variant=on  mask{zone=z.matrix_gains, gains=b.gains, subgain=4}
      mask init: same as building_PHPP_carnot83/BUILDING/ZONE_1/gain_1
      mask Display:
      | fprintf('GAINS:\n')
      | fprintf('\n%s', ga.name)
  infiltration_1 : Subsystem  Variant=on  mask{zone=z.matrix_wi, window=1}
      mask init: same as building_PHPP_carnot83/BUILDING/ZONE_1/infiltration_1
      mask Display:
      | fprintf('INFILTRATION:\n')
      | %fprintf('\n%s', const.name)
  infiltration_2 : Subsystem  Variant=on  mask{zone=z.matrix_wi, window=2}
      mask init: same as building_PHPP_carnot83/BUILDING/ZONE_1/infiltration_1
      mask Display:
      | fprintf('INFILTRATION:\n')
      | %fprintf('\n%s', const.name)
  infiltration_3 : Subsystem  Variant=on  mask{zone=z.matrix_wi, window=3}
      mask init: same as building_PHPP_carnot83/BUILDING/ZONE_1/infiltration_1
      mask Display:
      | fprintf('INFILTRATION:\n')
      | %fprintf('\n%s', const.name)
  infiltration_4 : Subsystem  Variant=on  mask{zone=z.matrix_wi, window=4}
      mask init: same as building_PHPP_carnot83/BUILDING/ZONE_1/infiltration_1
      mask Display:
      | fprintf('INFILTRATION:\n')
      | %fprintf('\n%s', const.name)
  infiltration_5 : Subsystem  Variant=on  mask{zone=z.matrix_wi, window=5}
      mask init: same as building_PHPP_carnot83/BUILDING/ZONE_1/infiltration_1
      mask Display:
      | fprintf('INFILTRATION:\n')
      | %fprintf('\n%s', const.name)
  room_node : Subsystem  Variant=on
  wall_1 : Subsystem  Variant=on  mask{zone=z.matrix_wd, construction=b.construction, wall=1}
      mask init: same as building_PHPP_carnot83/BUILDING/ZONE_1/wall_1
      mask Display:
      | fprintf('CONSTRUCTION:\n')
      | fprintf('\n%s', const.name)
  wall_2 : Subsystem  Variant=on  mask{zone=z.matrix_wd, construction=b.construction, wall=2}
      mask init: same as building_PHPP_carnot83/BUILDING/ZONE_1/wall_1
      mask Display:
      | fprintf('CONSTRUCTION:\n')
      | fprintf('\n%s', const.name)
  wall_3 : Subsystem  Variant=on  mask{zone=z.matrix_wd, construction=b.construction, wall=3}
      mask init: same as building_PHPP_carnot83/BUILDING/ZONE_1/wall_1
      mask Display:
      | fprintf('CONSTRUCTION:\n')
      | fprintf('\n%s', const.name)
  wall_4 : Subsystem  Variant=on  mask{zone=z.matrix_wd, construction=b.construction, wall=4}
      mask init: same as building_PHPP_carnot83/BUILDING/ZONE_1/wall_1
      mask Display:
      | fprintf('CONSTRUCTION:\n')
      | fprintf('\n%s', const.name)
  wall_5 : Subsystem  Variant=on  mask{zone=z.matrix_wd, construction=b.construction, wall=5}
      mask init: same as building_PHPP_carnot83/BUILDING/ZONE_1/wall_1
      mask Display:
      | fprintf('CONSTRUCTION:\n')
      | fprintf('\n%s', const.name)
  wall_6 : Subsystem  Variant=on  mask{zone=z.matrix_wd, construction=b.construction, wall=6}
      mask init: same as building_PHPP_carnot83/BUILDING/ZONE_1/wall_1
      mask Display:
      | fprintf('CONSTRUCTION:\n')
      | fprintf('\n%s', const.name)
  window_1 : Subsystem  Variant=on  mask{zone=z.matrix_wi, construction=b.construction, window=1}
      mask init: same as building_PHPP_carnot83/BUILDING/ZONE_1/window_1
      mask Display:
      | fprintf('CONSTRUCTION:\n')
      | fprintf('\n%s', const.name)
  window_2 : Subsystem  Variant=on  mask{zone=z.matrix_wi, construction=b.construction, window=2}
      mask init: same as building_PHPP_carnot83/BUILDING/ZONE_1/window_1
      mask Display:
      | fprintf('CONSTRUCTION:\n')
      | fprintf('\n%s', const.name)
  window_3 : Subsystem  Variant=on  mask{zone=z.matrix_wi, construction=b.construction, window=3}
      mask init: same as building_PHPP_carnot83/BUILDING/ZONE_1/window_1
      mask Display:
      | fprintf('CONSTRUCTION:\n')
      | fprintf('\n%s', const.name)
  window_4 : Subsystem  Variant=on  mask{zone=z.matrix_wi, construction=b.construction, window=4}
      mask init: same as building_PHPP_carnot83/BUILDING/ZONE_1/window_1
      mask Display:
      | fprintf('CONSTRUCTION:\n')
      | fprintf('\n%s', const.name)
  window_5 : Subsystem  Variant=on  mask{zone=z.matrix_wi, construction=b.construction, window=5}
      mask init: same as building_PHPP_carnot83/BUILDING/ZONE_1/window_1
      mask Display:
      | fprintf('CONSTRUCTION:\n')
      | fprintf('\n%s', const.name)
  BDB : Outport  VectorParamsAs1DForOutWhenUnconnected=off
  AIB : Outport  Port=2  VectorParamsAs1DForOutWhenUnconnected=off
  theta_out : Outport  Port=3  VectorParamsAs1DForOutWhenUnconnected=off
  wires:
  WDB/1 -> wall_3/1(WDB), wall_4/1(WDB), wall_5/1(WDB), wall_6/1(WDB), window_1/1(WDB), window_4/1(WDB), infiltration_2/2(WDB), infiltration_3/2(WDB), infiltration_4/2(WDB), infiltration_5/2(WDB), infiltration_1/2(WDB), window_5/1(WDB), window_3/1(WDB), window_2/1(WDB), wall_2/1(WDB), wall_1/1(WDB)
  room_node/1(BDB) -> BDB/1
  S_in/1 -> Subsystem4/1(S1)
  Qdot_in/1 -> wall_1/5(Qdot_in), wall_3/5(Qdot_in), wall_4/5(Qdot_in), wall_6/5(Qdot_in), wall_5/5(Qdot_in), wall_2/5(Qdot_in)
  Subsystem4/1(Sout) -> room_node/1(sum([S]))
  room_node/3(Qdot_sol) -> wall_3/6(Qdot_sol), wall_4/6(Qdot_sol), wall_6/6(Qdot_sol), wall_5/6(Qdot_sol), wall_2/6(Qdot_sol), wall_1/6(Qdot_sol)
  wall_1/2(theta_out) -> [theta_out_1]
  control/1 -> gain_2/2(control), gain_3/2(control), infiltration_1/3(control), infiltration_2/3(control), infiltration_3/3(control), infiltration_4/3(control), infiltration_5/3(control), gain_5/2(control), gain_4/2(control), gain_1/2(control), window_5/3(control), window_4/3(control), window_3/3(control), window_2/3(control), window_1/3(control)
  room_node/2(AIB) -> AIB/1, wall_3/4(AIB), wall_4/4(AIB), wall_5/4(AIB), wall_6/4(AIB), gain_2/1(AIB), gain_3/1(AIB), infiltration_2/1(AIB), infiltration_3/1(AIB), infiltration_4/1(AIB), infiltration_5/1(AIB), infiltration_1/1(AIB), gain_5/1(AIB), gain_4/1(AIB), gain_1/1(AIB), window_5/2(AIB), window_4/2(AIB), window_3/2(AIB), window_2/2(AIB), window_1/2(AIB), wall_2/4(AIB), wall_1/4(AIB)
  Mux/1 -> theta_out/1
  [theta_out_1] -> Mux/1
  [theta_out_2] -> Mux/2
  [theta_out_10] -> Mux/10
  [theta_out_9] -> Mux/9
  [theta_out_8] -> Mux/8
  [theta_out_7] -> Mux/7
  [theta_out_6] -> Mux/6
  [theta_out_5] -> Mux/5
  [theta_out_4] -> Mux/4
  [theta_out_3] -> Mux/3
  wall_2/2(theta_out) -> [theta_out_2]
  GDB/1 -> wall_1/2(GDB), wall_3/2(GDB), wall_4/2(GDB), wall_6/2(GDB), wall_5/2(GDB), wall_2/2(GDB)
  wall_3/2(theta_out) -> [theta_out_3]
  wall_4/2(theta_out) -> [theta_out_4]
  wall_5/2(theta_out) -> [theta_out_5]
  wall_6/2(theta_out) -> [theta_out_6]
  NDB/1 -> wall_1/3(NDB), wall_3/3(NDB), wall_4/3(NDB), wall_6/3(NDB), wall_5/3(NDB), wall_2/3(NDB)
  wall_1/1("[S]") -> Subsystem/1(S1)
  wall_6/1("[S]") -> Subsystem/6(S6)
  wall_2/1("[S]") -> Subsystem/2(S2)
  wall_3/1("[S]") -> Subsystem/3(S3)
  wall_4/1("[S]") -> Subsystem/4(S4)
  wall_5/1("[S]") -> Subsystem/5(S5)
  window_1/1("[S]") -> Subsystem1/1(S1)
  window_5/1("[S]") -> Subsystem1/5(S5)
  window_2/1("[S]") -> Subsystem1/2(S2)
  window_3/1("[S]") -> Subsystem1/3(S3)
  window_4/1("[S]") -> Subsystem1/4(S4)
  gain_1/1("[S]") -> Subsystem2/1(S1)
  gain_5/1("[S]") -> Subsystem2/5(S5)
  gain_2/1("[S]") -> Subsystem2/2(S2)
  gain_3/1("[S]") -> Subsystem2/3(S3)
  gain_4/1("[S]") -> Subsystem2/4(S4)
  infiltration_1/1("[S]") -> Subsystem3/1(S1)
  infiltration_5/1("[S]") -> Subsystem3/5(S5)
  infiltration_4/1("[S]") -> Subsystem3/4(S4)
  infiltration_3/1("[S]") -> Subsystem3/3(S3)
  infiltration_2/1("[S]") -> Subsystem3/2(S2)
  Subsystem3/1(Sout) -> Subsystem4/5(S5)
  Subsystem/1(Sout) -> Subsystem4/2(S2)
  Subsystem1/1(Sout) -> Subsystem4/3(S3)
  Subsystem2/1(Sout) -> Subsystem4/4(S4)
